simulink model "AterragemILS"  (R2020a)
settings: Solver=VariableStepAuto  StartTime=0.0  StopTime=370  RelTol=1e-3
values from neighbouring files (symbols this model uses):
  A = [Ybb  Yp+W0/U0      Yr-1  (g*cos(tt0))/U0 ... (first row only)    [Aterragem_sematuadores.m]    (also in EKC39.m)
  absangle_wind = 20    [Aterragem_sematuadores.m]    (also in EKC39.m)
  act_t = 0.1    [dados_sensores.m]
  act_vmax = 1    [dados_sensores.m]
  B = [YdA      YdR ... (first row only)    [Aterragem_sematuadores.m]    (also in EKC39.m)
  bb0 = 0    [Aterragem_sematuadores.m]    (also in EKC39.m)
  C = eye(4)    [Aterragem_sematuadores.m]    (also in EKC39.m)
  D = zeros(4,2)    [Aterragem_sematuadores.m]    (also in EKC39.m)
  dda_max = 20 * deg    (= 0.349065850399)    [Aterragem_sematuadores.m]    (also in EKC39.m)
  ddr_max = 20 * deg    (= 0.349065850399)    [Aterragem_sematuadores.m]    (also in EKC39.m)
  f = 40    [dados_sensores.m]
  F = pinv(G)    [Aterragem_sematuadores.m]    (also in EKC39.m)
  k_interior = [k3(:,1:4)]    [Aterragem_sematuadores.m]    (also in EKC39.m)
  k_lambda = k3(2,5)    [Aterragem_sematuadores.m]    (also in EKC39.m)
  p0 = 0    [Aterragem_sematuadores.m]    (also in EKC39.m)
  phi0 = 0    [Aterragem_sematuadores.m]    (also in EKC39.m)
  r0 = 0    [Aterragem_sematuadores.m]    (also in EKC39.m)
  s1_k = (s1_outmax-s1_outmin)/(s1_inmax-s1_inmin)    (= 5.72957795131)    [dados_sensores.m]
  s1_offset = s1_outmax-s1_k*s1_inmax    (= 2.5)    [dados_sensores.m]
  s1_outmax = 5    [dados_sensores.m]
  s1_outmin = 0    [dados_sensores.m]
  s1_t_const = 0.01    [dados_sensores.m]
  s2_k = (s2_outmax-s2_outmin)/(s2_inmax-s2_inmin)    (= 3.43774677078)    [dados_sensores.m]
  s2_offset = s2_outmax-s2_k*s2_inmax    (= 0)    [dados_sensores.m]
  s2_outmax = 3    [dados_sensores.m]
  s2_outmin = -3    [dados_sensores.m]
  s3_k = (s3_outmax-s3_outmin)/(s3_inmax-s3_inmin)    (= 8.91267681315)    [dados_sensores.m]
  s3_offset = s3_outmax-s3_k*s3_inmax    (= 14)    [dados_sensores.m]
  s3_outmax = 28    [dados_sensores.m]
  s3_outmin = 0    [dados_sensores.m]
  s5_max = 150*10^-6    (= 0.00015)    [dados_sensores.m]
  s5_sensibilidade = 3.63*10^-6    (= 3.63e-06)    [dados_sensores.m]
  tt0 = gg0+aa0    (= 0.125140107368)    [Aterragem_sematuadores.m]    (also in EKC39.m)
  U0 = 79.2*kn    (= 40.7439648)    [Aterragem_sematuadores.m]    (also in EKC39.m)
  v_wind = 10    [Aterragem_sematuadores.m]    (also in EKC39.m)
libraries: simulink x4
settings Model: PacingRate=0.890000  Creator=vicen  LastModifiedBy=vicen

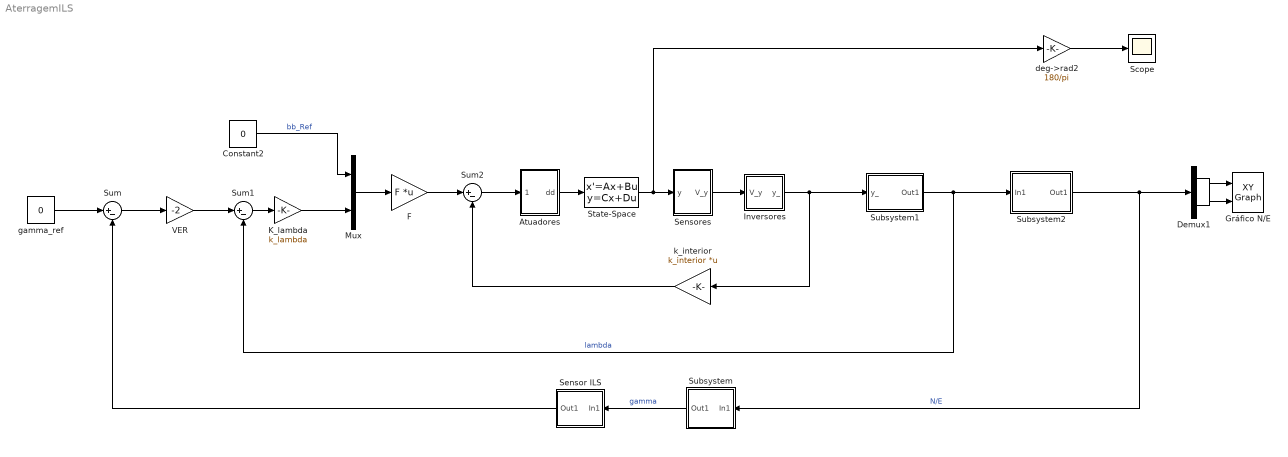
== system AterragemILS ==
  Atuadores : Subsystem
  Constant2 : Constant  Value=0
  Demux1 : Demux  Outputs=2
  F : Gain  Gain=F  Multiplication=Matrix(K*u)
  Gráfico N/E : simulink/Sinks/XY Graph  xmin=-1000  xmax=7800  ymin=-8000  ymax=1000  st=-1
  Inversores : Subsystem
  K_lambda : Gain  Gain=k_lambda
  Mux : Mux  Inputs=2
  Scope : Scope
  Sensor ILS : Subsystem
  Sensores : Subsystem
  State-Space : StateSpace  A=A  B=B  C=C  D=D  InitialCondition=0
  Subsystem : Subsystem
  Subsystem1 : Subsystem
  Subsystem2 : Subsystem
  Sum : Sum  Inputs=|+-
  Sum1 : Sum  Inputs=|+-
  Sum2 : Sum  Inputs=|+-
  VER : Gain  Gain=-2
  deg->rad2 : Gain  Gain=180/pi
  gamma_ref : Constant  Value=0
  k_interior : Gain  Gain=k_interior  Multiplication=Matrix(K*u)
  wires:
  Subsystem1/1(Out1) -> Subsystem2/1(In1), Sum1/2  "lambda"
  Constant2/1 -> Mux/1  "bb_Ref"
  K_lambda/1 -> Mux/2
  Sum/1 -> VER/1
  gamma_ref/1 -> Sum/1
  VER/1 -> Sum1/1
  Sum1/1 -> K_lambda/1
  Sensor ILS/1(Out1) -> Sum/2
  Subsystem2/1(Out1) -> Demux1/1, Subsystem/1(In1)  "N/E"
  Subsystem/1(Out1) -> Sensor ILS/1(In1)  "gamma"
  Sensores/1(V_y) -> Inversores/1(V_y)
  Sum2/1 -> Atuadores/1(V_dd)
  k_interior/1 -> Sum2/2
  Mux/1 -> F/1
  State-Space/1 -> deg->rad2/1, Sensores/1(y)
  F/1 -> Sum2/1
  Demux1/2 -> Gráfico N/E/1
  Demux1/1 -> Gráfico N/E/2
  Inversores/1(y_) -> k_interior/1, Subsystem1/1(y_)
  deg->rad2/1 -> Scope/1
  Atuadores/1(dd) -> State-Space/1

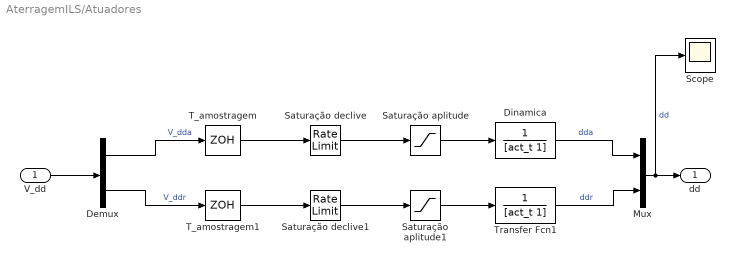
== system AterragemILS/Atuadores ==
  V_dd : Inport
  Demux : Demux  Outputs=2
  Dinamica : TransferFcn  Denominator=[act_t 1]
  Mux : Mux  Inputs=2
  Saturação aplitude : Saturate  UpperLimit=dda_max  LowerLimit=-dda_max
  Saturação aplitude1 : Saturate  UpperLimit=ddr_max  LowerLimit=-ddr_max
  Saturação declive : RateLimiter  RisingSlewLimit=act_vmax  FallingSlewLimit=-act_vmax  SampleTimeMode=inherited
  Saturação declive1 : RateLimiter  RisingSlewLimit=act_vmax  FallingSlewLimit=-act_vmax  SampleTimeMode=inherited
  Scope : Scope
  T_amostragem : ZeroOrderHold  SampleTime=1/f
  T_amostragem1 : ZeroOrderHold  SampleTime=1/f
  Transfer Fcn1 : TransferFcn  Denominator=[act_t 1]
  dd : Outport
  wires:
  Demux/1 -> T_amostragem/1  "V_dda"
  Demux/2 -> T_amostragem1/1  "V_ddr"
  Transfer Fcn1/1 -> Mux/2  "ddr"
  Mux/1 -> Scope/1, dd/1  "dd"
  V_dd/1 -> Demux/1
  Dinamica/1 -> Mux/1  "dda"
  Saturação declive/1 -> Saturação aplitude/1
  T_amostragem/1 -> Saturação declive/1
  T_amostragem1/1 -> Saturação declive1/1
  Saturação aplitude/1 -> Dinamica/1
  Saturação declive1/1 -> Saturação aplitude1/1
  Saturação aplitude1/1 -> Transfer Fcn1/1

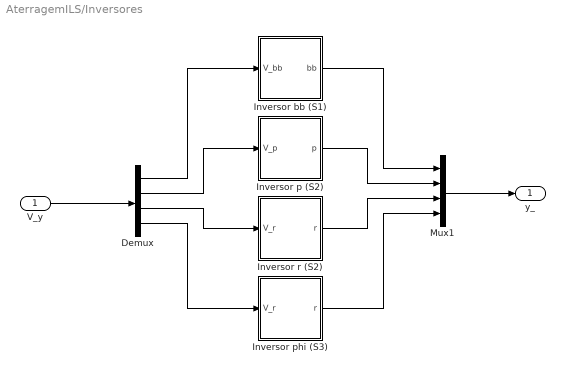
== system AterragemILS/Inversores ==
  V_y : Inport
  Demux : Demux
  Inversor bb (S1) : Subsystem
  Inversor p (S2) : Subsystem
  Inversor phi (S3) : Subsystem
  Inversor r (S2) : Subsystem
  Mux1 : Mux
  y_ : Outport
  wires:
  V_y/1 -> Demux/1
  Demux/2 -> Inversor p (S2)/1(V_p)
  Demux/4 -> Inversor phi (S3)/1(V_r)
  Demux/1 -> Inversor bb (S1)/1(V_bb)
  Inversor p (S2)/1(p) -> Mux1/2
  Inversor bb (S1)/1(bb) -> Mux1/1
  Mux1/1 -> y_/1
  Inversor r (S2)/1(r) -> Mux1/3
  Demux/3 -> Inversor r (S2)/1(V_r)
  Inversor phi (S3)/1(r) -> Mux1/4

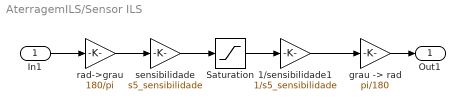
== system AterragemILS/Sensor ILS ==
  In1 : Inport
  1/sensibilidade1 : Gain  Gain=1/s5_sensibilidade
  Saturation : Saturate  UpperLimit=s5_max  LowerLimit=-s5_max
  "grau -> rad" : Gain  Gain=pi/180
  rad->grau : Gain  Gain=180/pi
  sensibilidade : Gain  Gain=s5_sensibilidade
  Out1 : Outport
  wires:
  In1/1 -> rad->grau/1
  rad->grau/1 -> sensibilidade/1
  sensibilidade/1 -> Saturation/1
  Saturation/1 -> 1/sensibilidade1/1
  1/sensibilidade1/1 -> "grau -> rad"/1
  "grau -> rad"/1 -> Out1/1

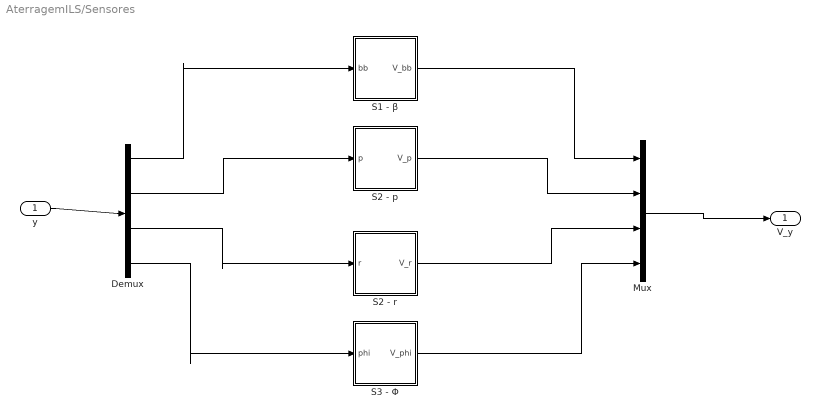
== system AterragemILS/Sensores ==
  y : Inport
  Demux : Demux
  Mux : Mux
  "S1 - β " : Subsystem
  S2 - p : Subsystem
  S2 - r : Subsystem
  S3 - Φ : Subsystem
  V_y : Outport
  wires:
  Mux/1 -> V_y/1
  "S1 - β "/1(V_bb) -> Mux/1
  S3 - Φ/1(V_phi) -> Mux/4
  S2 - p/1(V_p) -> Mux/2
  S2 - r/1(V_r) -> Mux/3
  y/1 -> Demux/1
  Demux/2 -> S2 - p/1(p)
  Demux/3 -> S2 - r/1(r)
  Demux/1 -> "S1 - β "/1(bb)
  Demux/4 -> S3 - Φ/1(phi)

== system AterragemILS/Subsystem ==
  In1 : Inport
  Demux : Demux  Outputs=2
  Divide : Product  Inputs=/*
  Trigonometric Function : Trigonometry  Operator=atan2
  Trigonometric Function1 : Trigonometry  Operator=atan
  Out1 : Outport
  wires:
  In1/1 -> Demux/1
  Demux/1 -> Divide/1  "N"
  Demux/2 -> Divide/2  "E"
  Divide/1 -> Trigonometric Function1/1
  Trigonometric Function1/1 -> Out1/1

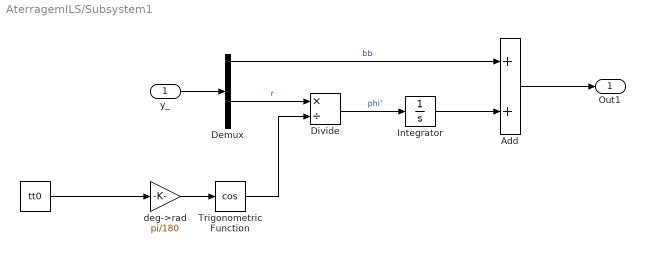
== system AterragemILS/Subsystem1 ==
  y_ : Inport
  " " : Constant  Value=tt0
  Add : Sum
  Demux : Demux
  Divide : Product  Inputs=*/
  Integrator : Integrator  InitialCondition=-pi/4
  Trigonometric Function : Trigonometry  Operator=cos
  deg->rad : Gain  Gain=pi/180
  Out1 : Outport
  wires:
  y_/1 -> Demux/1
  Demux/1 -> Add/1  "bb"
  Demux/3 -> Divide/1  "r"
  deg->rad/1 -> Trigonometric Function/1
  Trigonometric Function/1 -> Divide/2
  Divide/1 -> Integrator/1  "phi'"
  Integrator/1 -> Add/2
  Add/1 -> Out1/1
  " "/1 -> deg->rad/1

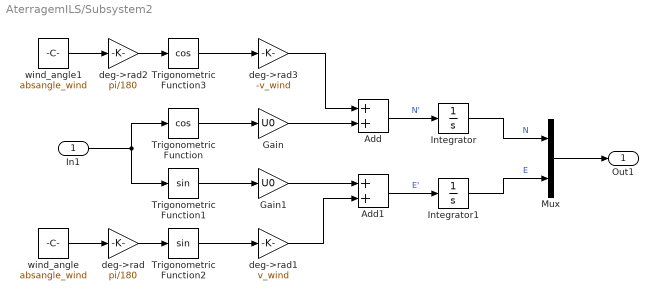
== system AterragemILS/Subsystem2 ==
  In1 : Inport
  Add : Sum
  Add1 : Sum
  Gain : Gain  Gain=U0
  Gain1 : Gain  Gain=U0
  Integrator : Integrator  InitialCondition=-7000
  Integrator1 : Integrator  InitialCondition=7000
  Mux : Mux  Inputs=2
  Trigonometric Function : Trigonometry  Operator=cos
  Trigonometric Function1 : Trigonometry
  Trigonometric Function2 : Trigonometry
  Trigonometric Function3 : Trigonometry  Operator=cos
  deg->rad : Gain  Gain=pi/180
  deg->rad1 : Gain  Gain=v_wind
  deg->rad2 : Gain  Gain=pi/180
  deg->rad3 : Gain  Gain=-v_wind
  wind_angle : Constant  Value=absangle_wind
  wind_angle1 : Constant  Value=absangle_wind
  Out1 : Outport
  wires:
  In1/1 -> Trigonometric Function1/1, Trigonometric Function/1
  Trigonometric Function/1 -> Gain/1
  Trigonometric Function1/1 -> Gain1/1
  Gain/1 -> Add/2
  Gain1/1 -> Add1/1
  wind_angle/1 -> deg->rad/1
  deg->rad/1 -> Trigonometric Function2/1
  Trigonometric Function2/1 -> deg->rad1/1
  deg->rad1/1 -> Add1/2
  deg->rad2/1 -> Trigonometric Function3/1
  wind_angle1/1 -> deg->rad2/1
  deg->rad3/1 -> Add/1
  Trigonometric Function3/1 -> deg->rad3/1
  Add1/1 -> Integrator1/1  "E'"
  Add/1 -> Integrator/1  "N'"
  Integrator1/1 -> Mux/2  "E"
  Integrator/1 -> Mux/1  "N"
  Mux/1 -> Out1/1

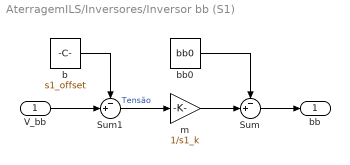
== system AterragemILS/Inversores/Inversor bb (S1) ==
  V_bb : Inport
  Sum : Sum  Inputs=-+|
  Sum1 : Sum  Inputs=-+|
  b : Constant  Value=s1_offset
  bb0 : Constant  Value=bb0
  m : Gain  Gain=1/s1_k
  bb : Outport
  wires:
  bb0/1 -> Sum/1
  b/1 -> Sum1/1
  V_bb/1 -> Sum1/2
  Sum1/1 -> m/1  "Tensão"
  m/1 -> Sum/2
  Sum/1 -> bb/1

== system AterragemILS/Inversores/Inversor p (S2) ==
  V_p : Inport
  Sum : Sum  Inputs=-+|
  Sum1 : Sum  Inputs=-+|
  b : Constant  Value=s2_offset
  bb0 : Constant  Value=p0
  m : Gain  Gain=1/s2_k
  p : Outport
  wires:
  bb0/1 -> Sum/1
  b/1 -> Sum1/1
  V_p/1 -> Sum1/2
  Sum1/1 -> m/1  "Tensão"
  m/1 -> Sum/2
  Sum/1 -> p/1

== system AterragemILS/Inversores/Inversor phi (S3) ==
  V_r : Inport
  Sum : Sum  Inputs=-+|
  Sum1 : Sum  Inputs=-+|
  b : Constant  Value=s3_offset
  bb0 : Constant  Value=phi0
  m : Gain  Gain=1/s3_k
  r : Outport
  wires:
  bb0/1 -> Sum/1
  b/1 -> Sum1/1
  V_r/1 -> Sum1/2
  Sum1/1 -> m/1  "Tensão"
  m/1 -> Sum/2
  Sum/1 -> r/1

== system AterragemILS/Inversores/Inversor r (S2) ==
  V_r : Inport
  Sum : Sum  Inputs=-+|
  Sum1 : Sum  Inputs=-+|
  b : Constant  Value=s2_offset
  bb0 : Constant  Value=r0
  m : Gain  Gain=1/s2_k
  r : Outport
  wires:
  bb0/1 -> Sum/1
  b/1 -> Sum1/1
  V_r/1 -> Sum1/2
  Sum1/1 -> m/1  "Tensão"
  m/1 -> Sum/2
  Sum/1 -> r/1

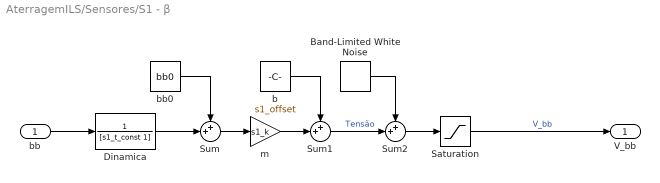
== system AterragemILS/Sensores/S1 - β  ==
  bb : Inport
  " Dinamica" : TransferFcn  Denominator=[s1_t_const 1]
  Band-Limited White Noise : simulink/Sources/Band-Limited White Noise  Cov=s1_power  Ts=1/f  seed=[23341]
  Saturation : Saturate  UpperLimit=s1_outmax  LowerLimit=s1_outmin
  Sum : Sum  Inputs=++|
  Sum1 : Sum  Inputs=++|
  Sum2 : Sum  Inputs=++|
  b : Constant  Value=s1_offset
  bb0 : Constant  Value=bb0
  m : Gain  Gain=s1_k
  V_bb : Outport
  wires:
  Sum2/1 -> Saturation/1
  bb/1 -> " Dinamica"/1
  bb0/1 -> Sum/1
  Sum/1 -> m/1
  Sum1/1 -> Sum2/2  "Tensão"
  m/1 -> Sum1/2
  b/1 -> Sum1/1
  Band-Limited White Noise/1 -> Sum2/1
  " Dinamica"/1 -> Sum/2
  Saturation/1 -> V_bb/1  "V_bb"

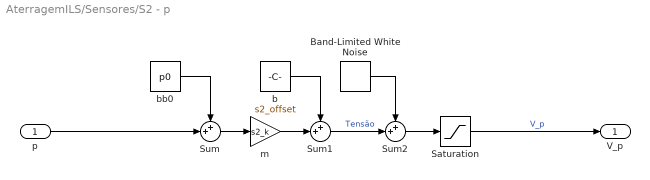
== system AterragemILS/Sensores/S2 - p ==
  p : Inport
  Band-Limited White Noise : simulink/Sources/Band-Limited White Noise  Cov=s2_power  Ts=1/f  seed=[01933]
  Saturation : Saturate  UpperLimit=s2_outmax  LowerLimit=s2_outmin
  Sum : Sum  Inputs=++|
  Sum1 : Sum  Inputs=++|
  Sum2 : Sum  Inputs=++|
  b : Constant  Value=s2_offset
  bb0 : Constant  Value=p0
  m : Gain  Gain=s2_k
  V_p : Outport
  wires:
  Sum2/1 -> Saturation/1
  bb0/1 -> Sum/1
  Sum/1 -> m/1
  Sum1/1 -> Sum2/2  "Tensão"
  m/1 -> Sum1/2
  b/1 -> Sum1/1
  Band-Limited White Noise/1 -> Sum2/1
  p/1 -> Sum/2
  Saturation/1 -> V_p/1  "V_p"

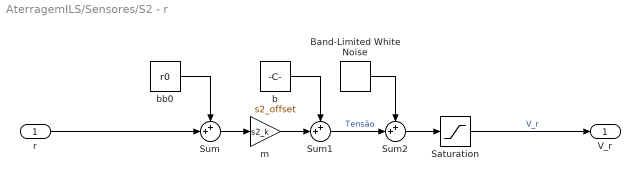
== system AterragemILS/Sensores/S2 - r ==
  r : Inport
  Band-Limited White Noise : simulink/Sources/Band-Limited White Noise  Cov=s2_power  Ts=1/f  seed=[26007]
  Saturation : Saturate  UpperLimit=s2_outmax  LowerLimit=s2_outmin
  Sum : Sum  Inputs=++|
  Sum1 : Sum  Inputs=++|
  Sum2 : Sum  Inputs=++|
  b : Constant  Value=s2_offset
  bb0 : Constant  Value=r0
  m : Gain  Gain=s2_k
  V_r : Outport
  wires:
  Sum2/1 -> Saturation/1
  bb0/1 -> Sum/1
  Sum/1 -> m/1
  Sum1/1 -> Sum2/2  "Tensão"
  m/1 -> Sum1/2
  b/1 -> Sum1/1
  Band-Limited White Noise/1 -> Sum2/1
  r/1 -> Sum/2
  Saturation/1 -> V_r/1  "V_r"

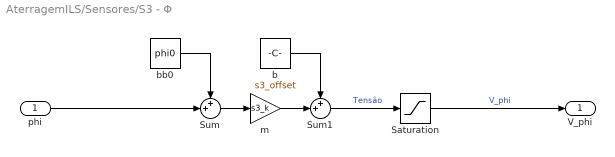
== system AterragemILS/Sensores/S3 - Φ ==
  phi : Inport
  Saturation : Saturate  UpperLimit=s3_outmax  LowerLimit=s3_outmin
  Sum : Sum  Inputs=++|
  Sum1 : Sum  Inputs=++|
  b : Constant  Value=s3_offset
  bb0 : Constant  Value=phi0
  m : Gain  Gain=s3_k
  V_phi : Outport
  wires:
  bb0/1 -> Sum/1
  Sum/1 -> m/1
  Sum1/1 -> Saturation/1  "Tensão"
  m/1 -> Sum1/2
  b/1 -> Sum1/1
  phi/1 -> Sum/2
  Saturation/1 -> V_phi/1  "V_phi"
